simulink model "simu"  (R2025b)
settings: Solver=ode1  StartTime=0.0  StopTime=Tstop  FixedStep=dt  RelTol=1e-3
values from neighbouring files (symbols this model uses):
  N = dim2 / 2    [animation1.m]    (also in cbf_centralized.m = 10; cbf_decentralized.m = 7; centralized_cbf_step.m = evalin('base', 'N'); hybrid_cbf_step.m = evalin('base','N'))
  v0_vec = reshape(v', [], 1)    [initialization.m]    (also in inizialize.m)
  x0_vec = reshape(x', [], 1)    [initialization.m]    (also in inizialize.m)
settings Model: Creator=Filippo  LastModifiedBy=Filippo
settings DataIOCC: ReturnWorkspaceOutputs=off

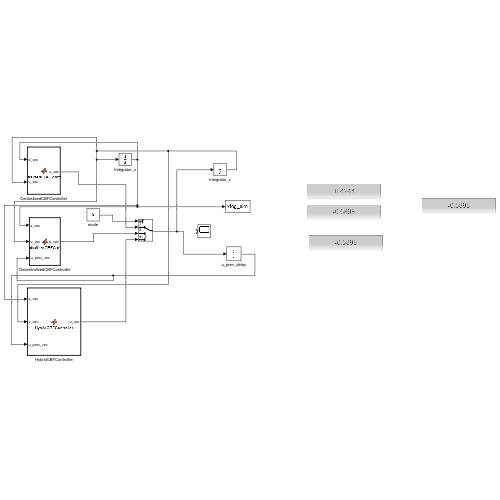
[thumbnail: Simulink's stored preview of the top-level diagram]
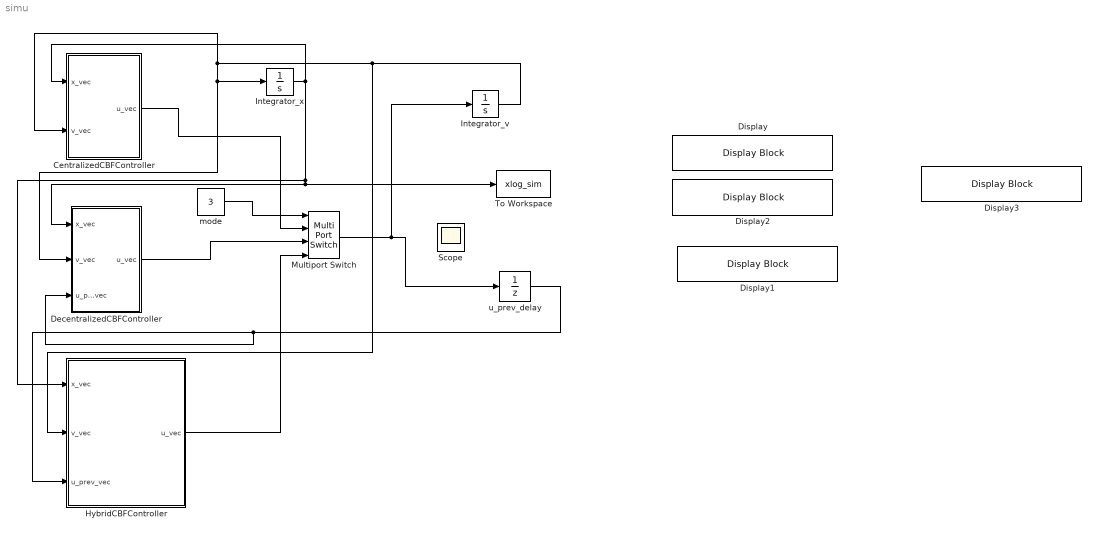
== system simu ==
  CentralizedCBFController : MATLAB Function  TreatAsAtomicUnit=on
  DecentralizedCBFController : MATLAB Function  TreatAsAtomicUnit=on
  Display{,1..3} (4 alike) : DisplayBlock  LabelPosition=Hide  Transparency=1  GridColor=[0.502, 0.502, 0.502]
  HybridCBFController : MATLAB Function  TreatAsAtomicUnit=on
  Integrator_v : Integrator  InitialCondition=v0_vec
  Integrator_x : Integrator  InitialCondition=x0_vec
  Multiport Switch : MultiPortSwitch  SaturateOnIntegerOverflow=off  InputSameDT=off
  Scope : Scope
      settings: ActiveDisplayYMinimum=-13.482569527528531  ActiveDisplayYMaximum=11.081645377721495
  To Workspace : ToWorkspace  VariableName=xlog_sim  SampleTime=-1
  mode : Constant  Value=3
  u_prev_delay : UnitDelay  InitialCondition=zeros(2*N,1)  SampleTime=-1  HasFrameUpgradeWarning=on
  wires:
  Integrator_v/1 -> HybridCBFController/2(v_vec), Integrator_x/1, DecentralizedCBFController/2(v_vec), CentralizedCBFController/2(v_vec)
  Integrator_x/1 -> CentralizedCBFController/1(x_vec), HybridCBFController/1(x_vec), DecentralizedCBFController/1(x_vec), To Workspace/1
  CentralizedCBFController/1(u_vec) -> Multiport Switch/2
  u_prev_delay/1 -> HybridCBFController/3(u_prev_vec), DecentralizedCBFController/3(u_prev_vec)
  mode/1 -> Multiport Switch/1
  HybridCBFController/1(u_vec) -> Multiport Switch/4
  Multiport Switch/1 -> Integrator_v/1, u_prev_delay/1
  DecentralizedCBFController/1(u_vec) -> Multiport Switch/3

== matlab function simu/CentralizedCBFController ==
  data: x_vec input; u_vec output; v_vec input
function u_vec = CentralizedCBFController(x_vec, v_vec)
%#codegen
% Wrapper per chiamare la funzione esterna centralized_cbf_step
% dallo schema Simulink.

    coder.extrinsic('centralized_cbf_step');   % dico al coder che è una funzione MATLAB "normale"

    % Per permettere a Simulink di capire le dimensioni, prealloca u_vec
    % N = 5 --> 2N = 10. Se vuoi usare N dal workspace:
    %   coder.extrinsic('evalin');
    %   N = evalin('base','N');
    %   u_vec = zeros(2*N,1);
    N = 5;              % <-- se ora stai lavorando con 5 robot
    u_vec = zeros(2*N,1);

    % Chiamata vera e propria alla funzione di controllo
    u_vec = centralized_cbf_step(x_vec, v_vec);
end

== matlab function simu/HybridCBFController ==
  data: x_vec input; u_vec output; v_vec input; u_prev_vec input
function u_vec = HybridCBFController(x_vec, v_vec, u_prev_vec)
%#codegen
% Wrapper per hybrid_cbf_step.m

coder.extrinsic('hybrid_cbf_step');

% per inferenza dimensioni
N = 5;              % oppure leggi dal base workspace con evalin se vuoi
u_vec = zeros(2*N,1);

u_vec = hybrid_cbf_step(x_vec, v_vec, u_prev_vec);
end

== matlab function simu/DecentralizedCBFController ==
  data: x_vec input; u_vec output; v_vec input; u_prev_vec input
function u_vec = DecentralizedCBFController(x_vec, v_vec, u_prev_vec)
%#codegen
% Wrapper per chiamare decentralized_cbf_step da Simulink

coder.extrinsic('decentralized_cbf_step');

% Numero agenti (qui puoi fissare N=5 o leggere dal base workspace)
N = 5;                     % oppure usa evalin se vuoi:
% coder.extrinsic('evalin');
% N = evalin('base','N');

u_vec = zeros(2*N,1);      % per inferenza dimensioni

u_vec = decentralized_cbf_step(x_vec, v_vec, u_prev_vec);
end
